simulink library "examplePlant_cl"  (R2018b)
settings: Solver=VariableStepAuto  StartTime=0.0  StopTime=10.0  RelTol=1e-3
settings Model: Creator=mcobb  LastModifiedBy=mcobb

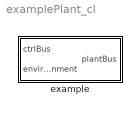
== system examplePlant_cl ==
  example : Subsystem

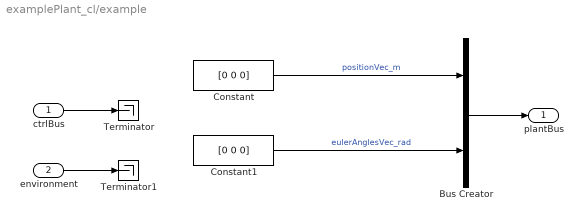
== system examplePlant_cl/example ==
  ctrlBus : Inport  OutDataTypeStr=Bus: ctrlBus
  environment : Inport  Port=2  OutDataTypeStr=Bus: envBus
  Bus Creator : BusCreator  Inputs=2
  Constant : Constant  Value=[0 0 0]
  Constant1 : Constant  Value=[0 0 0]
  Terminator : Terminator
  Terminator1 : Terminator
  plantBus : Outport  OutDataTypeStr=Bus: plantBus
  wires:
  Bus Creator/1 -> plantBus/1
  Constant/1 -> Bus Creator/1  "positionVec_m"
  Constant1/1 -> Bus Creator/2  "eulerAnglesVec_rad"
  ctrlBus/1 -> Terminator/1
  environment/1 -> Terminator1/1
